simulink subsystem "refuel_GS_subsystem"  (R2025a)
settings: Solver=VariableStepAuto  StartTime=0.0  StopTime=10.0  RelTol=1e-3
settings Model: Creator=MW  LastModifiedBy=MW

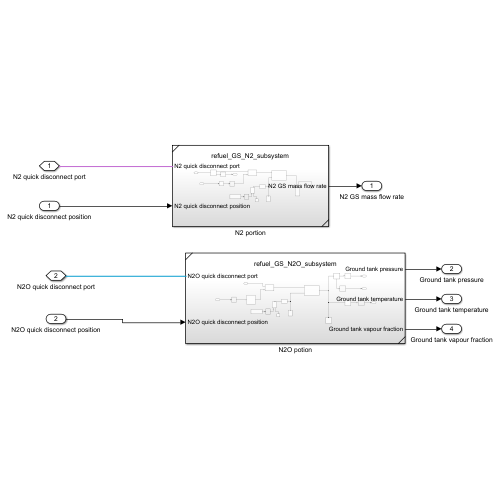
[thumbnail: Simulink's stored preview of the top-level diagram]
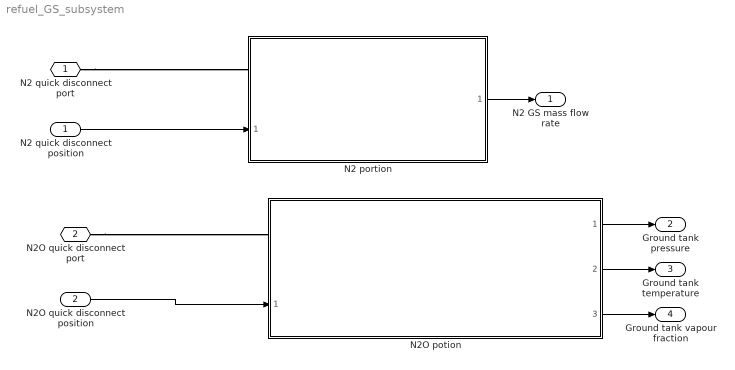
== system refuel_GS_subsystem ==
  N2 quick disconnect position : Inport
  N2O quick disconnect position : Inport  Port=2
  N2 portion : Subsystem  ReferencedSubsystem=refuel_GS_N2_subsystem
      settings: PortSchema="{\"entries\":[{\"content\":{\"sides\":[{\"content\":{\"connectorIds\":[\"LConn1\",\"In1\"]},\"type\":\"ConnectorPlacement.EquallySpacedRectSide\",\"uuid\":\"80a1b4a4-a86f-460b-b4b9-f1e834cc0a6f\"},{\"content\":{\"connectorIds\":[\"Out1\"],\"side\":\"RIGHT\"},\"type\":\"ConnectorPlacement.EquallySpacedRectSide\",\"uuid\":\"7a691a14-4b0a-4077-9abf-8e4fa479ec3d\"},{\"content\":{\"side\":\"TOP\"},\"type\":\"ConnectorPlacement.EquallySpacedRectSide\",\"uuid\":\"b8dd7e20-acb6-44c1-83ed-0b89a390ff72\"}]},\"type\":\"ConnectorPlacement.EquallySpacedConnector\",\"uuid\":\"2e88b817-b41b-4786-aed1-deff05c2a84d\"}],\"packageUris\":[\"http://schema.mathworks.com/mf0/Connector/R2020b\"],\"version\":\"1.0\"}"
  N2O potion : Subsystem  ReferencedSubsystem=refuel_GS_N2O_subsystem
      settings: PortSchema="{\"entries\":[{\"content\":{\"sides\":[{\"content\":{\"connectorIds\":[\"LConn1\",\"In1\"]},\"type\":\"ConnectorPlacement.EquallySpacedRectSide\",\"uuid\":\"80a1b4a4-a86f-460b-b4b9-f1e834cc0a6f\"},{\"content\":{\"connectorIds\":[\"Out1\",\"Out2\",\"Out3\"],\"side\":\"RIGHT\"},\"type\":\"ConnectorPlacement.EquallySpacedRectSide\",\"uuid\":\"7a691a14-4b0a-4077-9abf-8e4fa479ec3d\"},{\"content\":{\"side\":\"TOP\"},\"type\":\"ConnectorPlacement.EquallySpacedRectSide\",\"uuid\":\"b8dd7e20-acb6-44c1-83ed-0b89a390ff72\"}]},\"type\":\"ConnectorPlacement.EquallySpacedConnector\",\"uuid\":\"2e88b817-b41b-4786-aed1-deff05c2a84d\"}],\"packageUris\":[\"http://schema.mathworks.com/mf0/Connector/R2020b\"],\"version\":\"1.0\"}"
  N2 quick disconnect port : PMIOPort  Side=Left
  N2O quick disconnect port : PMIOPort  Port=2  Side=Left
  N2 GS mass flow rate : Outport
  Ground tank pressure : Outport  Port=2
  Ground tank temperature : Outport  Port=3
  Ground tank vapour fraction : Outport  Port=4
  wires:
  N2 quick disconnect position/1 -> N2 portion/1
  N2O quick disconnect position/1 -> N2O potion/1
  N2 portion/1 -> N2 GS mass flow rate/1
  N2O potion/1 -> Ground tank pressure/1
  N2O potion/2 -> Ground tank temperature/1
  N2O potion/3 -> Ground tank vapour fraction/1
  connections:
  N2O quick disconnect port/RConn1 -- N2O potion/LConn1
  N2 quick disconnect port/RConn1 -- N2 portion/LConn1
